simulink model "rst_auto_reg_complete_2018a"  (R2018a)
settings: Solver=VariableStepAuto  StartTime=0.0  StopTime=100  RelTol=1e-3
undefined symbols (not defined in the file): A, B, ep, initial_theta, Ta, Tas, theta_switch_time, Ts, w0
libraries: dspinverses x6, simulink x1
settings Model: Creator=tarci  LastModifiedBy=tarci

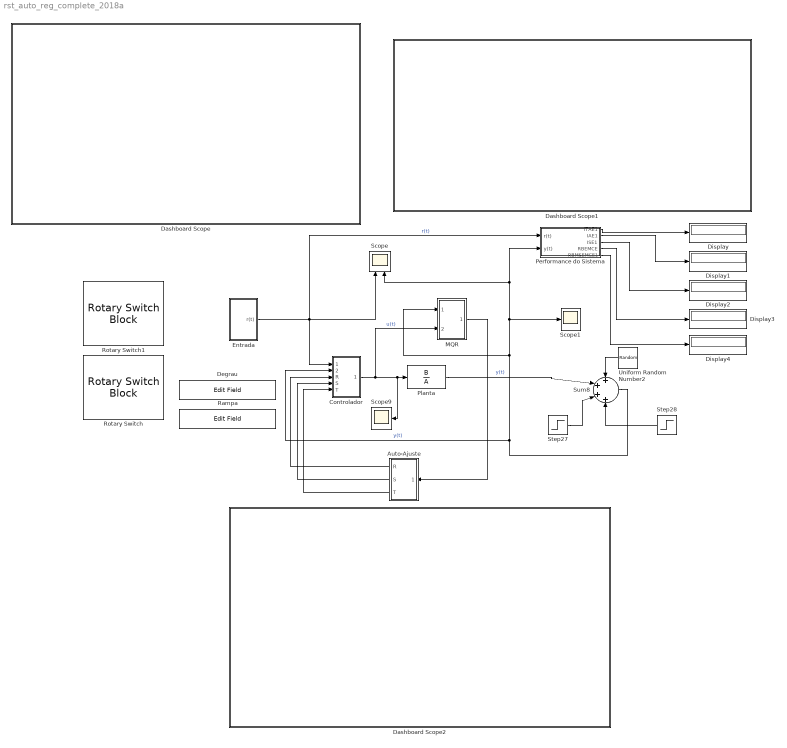
== system rst_auto_reg_complete_2018a ==
  Auto-Ajuste : Subsystem
  Controlador : Subsystem
  Dashboard Scope : Subsystem  DialogController=hmiCreateDDGDialog  IsWebBlock=on  mask(MWDashboardBlock){webBlockId=9b3c1e76-0f89-451d-9ebf-e152fc28c02b, webBlockType=sdiscope, ShowInitialText=on, HMISrcModelName=rst_auto_reg_complete_2018a}
      mask prompts: webBlockId "WebBlock Id"; webBlockType "WebBlock Type"; HMISrcModelName "Source Model"
      mask help: SimulinkHMI:dialogs:HMIScopeDialogDesc
      mask Help: helpview([docroot '/mapfiles/simulink.map'], 'hmi_scope')
      mask Display:
      | if strcmp(get_param(bdroot(gcb),'BlockDiagramType'), 'library')
      |     image([(matlabroot) '/toolbox/simulink/hmi/icons/DashboardScope.png']);
      | end
  Dashboard Scope1 : Subsystem  DialogController=hmiCreateDDGDialog  IsWebBlock=on  mask(MWDashboardBlock){webBlockId=06d563f5-1f97-498a-bfac-7182b92c07c4, webBlockType=sdiscope, ShowInitialText=on, HMISrcModelName=rst_auto_reg_complete_2018a}
      mask prompts: webBlockId "WebBlock Id"; webBlockType "WebBlock Type"; HMISrcModelName "Source Model"
      mask help: SimulinkHMI:dialogs:HMIScopeDialogDesc
      mask Help: helpview([docroot '/mapfiles/simulink.map'], 'hmi_scope')
      mask Display:
      | if strcmp(get_param(bdroot(gcb),'BlockDiagramType'), 'library')
      |     image([(matlabroot) '/toolbox/simulink/hmi/icons/DashboardScope.png']);
      | end
  Dashboard Scope2 : Subsystem  DialogController=hmiCreateDDGDialog  IsWebBlock=on  mask(MWDashboardBlock){webBlockId=9828eeca-fbfb-4c59-aa67-bf465e2bb125, webBlockType=sdiscope, ShowInitialText=on, HMISrcModelName=rst_auto_reg_complete_2018a}
      mask prompts: webBlockId "WebBlock Id"; webBlockType "WebBlock Type"; HMISrcModelName "Source Model"
      mask help: SimulinkHMI:dialogs:HMIScopeDialogDesc
      mask Help: helpview([docroot '/mapfiles/simulink.map'], 'hmi_scope')
      mask Display:
      | if strcmp(get_param(bdroot(gcb),'BlockDiagramType'), 'library')
      |     image([(matlabroot) '/toolbox/simulink/hmi/icons/DashboardScope.png']);
      | end
  Degrau : EditField  WebBlockId=626  LabelPosition=Hide  Alignment=Center
  Display{,1..4} (5 alike) : Display
  Entrada : Subsystem
  MQR : Subsystem
  Performance do Sistema : Subsystem
  Planta : DiscreteFilter  Numerator=B  Denominator=A  SampleTime=Ta  a0EqualsOne=on
  Rampa : EditField  WebBlockId=627  LabelPosition=Hide  Alignment=Center
  Rotary Switch : RotarySwitchBlock  WebBlockId=461
      settings: Values={{'Degrau', 'Rampa', 'Senoide'}, [1 2 3]}
  Rotary Switch1 : RotarySwitchBlock  WebBlockId=519
      settings: Values={{'Degrau', 'Rampa', 'Senoide'}, [1 2 3]}
  Scope : Scope  NumInputPorts=2
  Scope1 : Scope
  Scope9 : Scope
  Step27 : Step  Time=90  SampleTime=0
  Step28 : Step  Time=91  After=-1  SampleTime=0
  Sum8 : Sum  Inputs=++++
  Uniform Random Number2 : UniformRandomNumber  Minimum=-0.1  Maximum=0.1  SampleTime=0
  wires:
  Sum8/1 -> Controlador/2(y(t)), Scope1/1, Performance do Sistema/2(y(t)), Scope/2, MQR/1(y(t))  "y(t)"
  Step28/1 -> Sum8/4
  Planta/1 -> Sum8/2  "y(t)"
  Step27/1 -> Sum8/3
  Uniform Random Number2/1 -> Sum8/1
  MQR/1("Theta(t) ") -> Auto-Ajuste/1(Theta)
  Controlador/1(u(t)) -> Scope9/1, Planta/1, MQR/2("u(t) ")  "u(t)"
  Auto-Ajuste/1(R) -> Controlador/3(R)
  Auto-Ajuste/2(S) -> Controlador/4(S)
  Auto-Ajuste/3(T) -> Controlador/5(T)
  Entrada/1(r(t)) -> Performance do Sistema/1(r(t)), Scope/1, Controlador/1(r(t))  "r(t)"
  Performance do Sistema/1(ITAE1) -> Display/1
  Performance do Sistema/2(IAE1) -> Display1/1
  Performance do Sistema/3(ISE1) -> Display2/1
  Performance do Sistema/4(RBEMCE) -> Display3/1
  Performance do Sistema/5(RBMSEMCE1) -> Display4/1

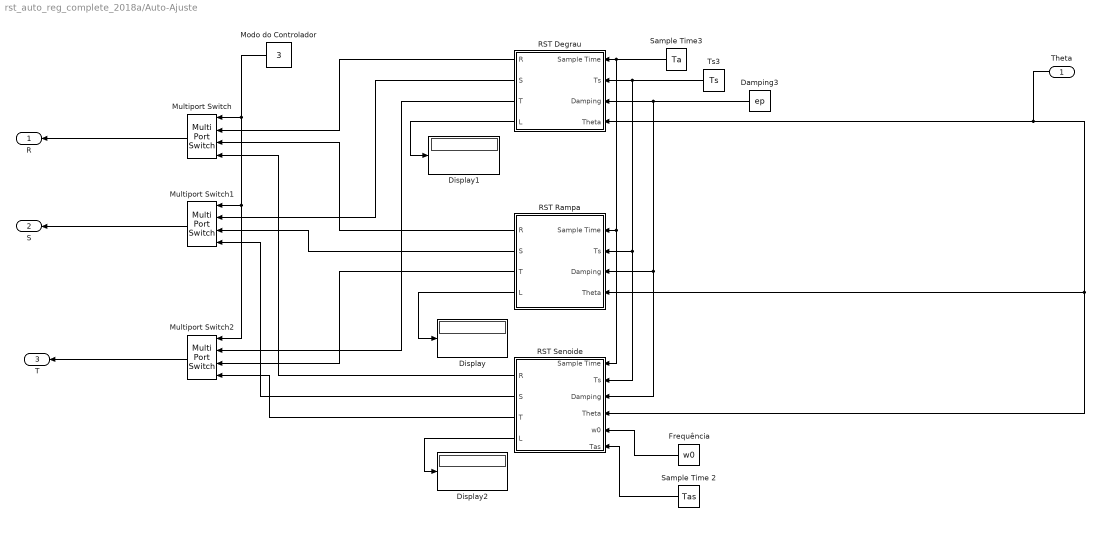
== system rst_auto_reg_complete_2018a/Auto-Ajuste ==
  Theta : Inport
  Damping3 : Constant  Value=ep
  Display : Display
  Display1 : Display
  Display2 : Display
  Frequência : Constant  Value=w0
  Modo do Controlador : Constant  Value=3
  Multiport Switch : MultiPortSwitch
  Multiport Switch1 : MultiPortSwitch
  Multiport Switch2 : MultiPortSwitch
  RST Degrau : Subsystem
  RST Rampa : Subsystem
  RST Senoide : Subsystem
  Sample Time 2 : Constant  Value=Tas
  Sample Time3 : Constant  Value=Ta
  Ts3 : Constant  Value=Ts
  R : Outport
  S : Outport  Port=2
  T : Outport  Port=3
  wires:
  Modo do Controlador/1 -> Multiport Switch2/1, Multiport Switch1/1, Multiport Switch/1
  RST Degrau/1(R) -> Multiport Switch/2
  Damping3/1 -> RST Senoide/3(Damping), RST Rampa/3(Damping), RST Degrau/3(Damping)
  RST Degrau/3(T) -> Multiport Switch2/2
  Theta/1 -> RST Senoide/4(Theta), RST Rampa/4(Theta), RST Degrau/4(Theta)
  RST Rampa/3(T) -> Multiport Switch2/3
  Sample Time3/1 -> RST Senoide/1(Sample Time), RST Rampa/1(Sample Time), RST Degrau/1(Sample Time)
  Sample Time 2/1 -> RST Senoide/6(Tas)
  Frequência/1 -> RST Senoide/5(w0)
  RST Rampa/1(R) -> Multiport Switch/3
  RST Senoide/2(S) -> Multiport Switch1/4
  RST Degrau/2(S) -> Multiport Switch1/2
  Ts3/1 -> RST Senoide/2(Ts), RST Rampa/2(Ts), RST Degrau/2(Ts)
  RST Senoide/1(R) -> Multiport Switch/4
  Multiport Switch/1 -> R/1
  Multiport Switch1/1 -> S/1
  Multiport Switch2/1 -> T/1
  RST Rampa/4(L) -> Display/1
  RST Senoide/3(T) -> Multiport Switch2/4
  RST Rampa/2(S) -> Multiport Switch1/3
  RST Degrau/4(L) -> Display1/1
  RST Senoide/4(L) -> Display2/1

== system rst_auto_reg_complete_2018a/Controlador ==
  r(t) : Inport
  y(t) : Inport  Port=2
  R : Inport  Port=3
  S : Inport  Port=4
  T : Inport  Port=5
  1/S3 : DiscreteFilter  Numerator=1  DenominatorSource=Input port  Denominator=1  SampleTime=Ta  a0EqualsOne=on
      settings: InputPortMap=u0,p3
  R3 : DiscreteFilter  NumeratorSource=Input port  Numerator=[-620.2 131.3]  Denominator=1  SampleTime=Ta
      settings: InputPortMap=u0,p1
  Sum11 : Sum  Inputs=|+-
  T3 : DiscreteFilter  NumeratorSource=Input port  Numerator=13.39  Denominator=1  SampleTime=Ta
      settings: InputPortMap=u0,p1
  u(t) : Outport
  wires:
  T3/1 -> Sum11/1
  T/1 -> T3/2  "T"
  Sum11/1 -> 1/S3/1
  R3/1 -> Sum11/2
  R/1 -> R3/2
  S/1 -> 1/S3/2
  r(t)/1 -> T3/1
  y(t)/1 -> R3/1
  1/S3/1 -> u(t)/1  "u(t)"

== system rst_auto_reg_complete_2018a/Dashboard Scope ==

== system rst_auto_reg_complete_2018a/Dashboard Scope1 ==

== system rst_auto_reg_complete_2018a/Dashboard Scope2 ==

== system rst_auto_reg_complete_2018a/Entrada ==
  Multiport Switch : MultiPortSwitch
  Ramp : simulink/Sources/Ramp  slope=1  start=0  InitialOutput=0
  Sine Wave : Sin  Frequency=w0  SampleTime=Tas
  Step1 : Step  Time=0  After=2  SampleTime=0
  Tipo de Entrada : Constant  Value=3
  r(t) : Outport
  wires:
  Sine Wave/1 -> Multiport Switch/4
  Step1/1 -> Multiport Switch/2
  Ramp/1 -> Multiport Switch/3
  Tipo de Entrada/1 -> Multiport Switch/1
  Multiport Switch/1 -> r(t)/1

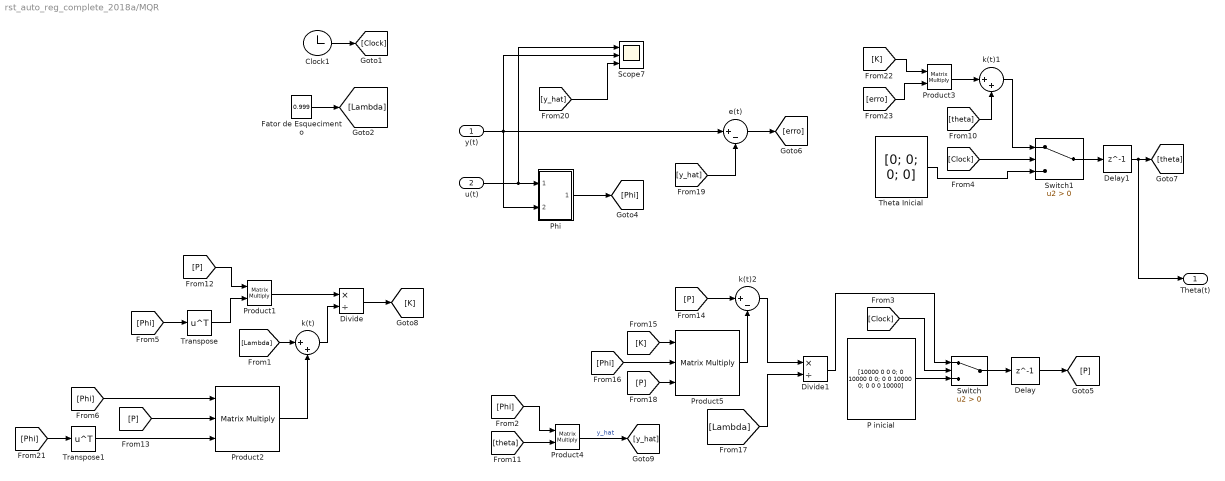
== system rst_auto_reg_complete_2018a/MQR ==
  y(t) : Inport
  "u(t) " : Inport  Port=2
  Clock1 : Clock
  Delay : Delay  DelayLength=1  InitialCondition=0
  Delay1 : Delay  DelayLength=1  InitialCondition=0
  Divide : Product  Inputs=*/
  Divide1 : Product  Inputs=*/
  "Fator de Esquecimento " : Constant  Value=0.999
  P inicial : Constant  Value=[10000 0 0 0; 0 10000 0 0; 0 0 10000 0; 0 0 0 10000]
  Phi : Subsystem
  Product1 : Product  Multiplication=Matrix(*)
  Product2 : Product  Inputs=3  Multiplication=Matrix(*)
  Product3 : Product  Multiplication=Matrix(*)
  Product4 : Product  Multiplication=Matrix(*)
  Product5 : Product  Inputs=3  Multiplication=Matrix(*)
  Scope7 : Scope  NumInputPorts=3
  Switch : Switch  Criteria=u2 > Threshold
  Switch1 : Switch  Criteria=u2 > Threshold
  "Theta Inicial " : Constant  Value=[0; 0; 0; 0]
  Transpose : Math  Operator=transpose  SaturateOnIntegerOverflow=on
  Transpose1 : Math  Operator=transpose  SaturateOnIntegerOverflow=on
  e(t) : Sum  Inputs=|+-
  k(t) : Sum  Inputs=|++
  k(t)1 : Sum  Inputs=|++
  k(t)2 : Sum  Inputs=|+-
  "Theta(t) " : Outport
  wires:
  k(t)/1 -> Divide/2
  [Phi] -> Product4/1
  Phi/1(Phi) -> [Phi]
  k(t)1/1 -> Switch1/1
  [y_hat] -> Scope7/3
  Switch1/1 -> Delay1/1
  [K] -> Product3/1
  Product2/1 -> k(t)/2
  [Clock] -> Switch1/2
  y(t)/1 -> e(t)/1, Scope7/2, Phi/2(y(t))
  k(t)2/1 -> Divide1/1
  Delay1/1 -> "Theta(t) "/1, [theta]
  Product5/1 -> k(t)2/2
  "u(t) "/1 -> Scope7/1, Phi/1(u(t))
  Switch/1 -> Delay/1
  [Lambda] -> Divide1/2
  Product1/1 -> Divide/1
  e(t)/1 -> [erro]
  Product3/1 -> k(t)1/1
  Delay/1 -> [P]
  [Phi] -> Transpose1/1
  [P] -> Product5/3
  "Fator de Esquecimento "/1 -> [Lambda]
  "Theta Inicial "/1 -> Switch1/3
  Transpose1/1 -> Product2/3
  Divide1/1 -> Switch/1
  [Phi] -> Transpose/1
  [Clock] -> Switch/2
  [theta] -> Product4/2
  [P] -> k(t)2/1
  [theta] -> k(t)1/2
  [P] -> Product2/2
  [Lambda] -> k(t)/1
  Transpose/1 -> Product1/2
  Clock1/1 -> [Clock]
  [erro] -> Product3/2
  [y_hat] -> e(t)/2
  [K] -> Product5/1
  P inicial/1 -> Switch/3
  [P] -> Product1/1
  [Phi] -> Product2/1
  Divide/1 -> [K]
  [Phi] -> Product5/2
  Product4/1 -> [y_hat]  "y_hat"

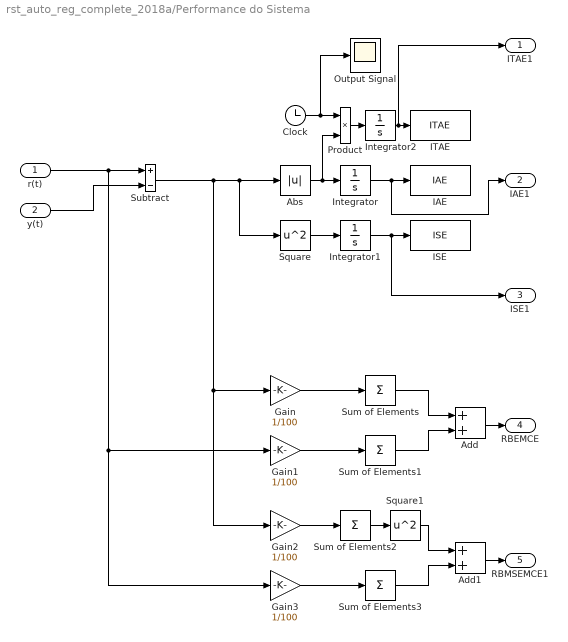
== system rst_auto_reg_complete_2018a/Performance do Sistema ==
  r(t) : Inport
  y(t) : Inport  Port=2
  Abs : Abs
  Add : Sum
  Add1 : Sum
  Clock : Clock
  Gain{,1..3} (4 alike) : Gain  Gain=1/100
  IAE : ToWorkspace  VariableName=IAE  SaveFormat=Timeseries  SampleTime=-1
  ISE : ToWorkspace  VariableName=ISE  SaveFormat=Timeseries  SampleTime=-1
  ITAE : ToWorkspace  VariableName=ITAE  SaveFormat=Timeseries  SampleTime=-1
  Integrator : Integrator
  Integrator1 : Integrator
  Integrator2 : Integrator
  Output Signal : Scope
  Product : Product
  Square : Math  Operator=square  SaturateOnIntegerOverflow=on
  Square1 : Math  Operator=square  SaturateOnIntegerOverflow=on
  Subtract : Sum  Inputs=+-
  Sum of Elements{,1..3} (4 alike) : Sum  Inputs=+
  ITAE1 : Outport
  IAE1 : Outport  Port=2
  ISE1 : Outport  Port=3
  RBEMCE : Outport  Port=4
  RBMSEMCE1 : Outport  Port=5
  wires:
  y(t)/1 -> Subtract/2
  Abs/1 -> Product/2, Integrator/1
  Integrator/1 -> IAE1/1, IAE/1
  Integrator1/1 -> ISE1/1, ISE/1
  Square/1 -> Integrator1/1
  Clock/1 -> Output Signal/1, Product/1
  Product/1 -> Integrator2/1
  Integrator2/1 -> ITAE1/1, ITAE/1
  Gain/1 -> Sum of Elements/1
  Gain1/1 -> Sum of Elements1/1
  Sum of Elements/1 -> Add/1
  Sum of Elements1/1 -> Add/2
  Add/1 -> RBEMCE/1
  Add1/1 -> RBMSEMCE1/1
  Sum of Elements3/1 -> Add1/2
  Sum of Elements2/1 -> Square1/1
  Gain3/1 -> Sum of Elements3/1
  Gain2/1 -> Sum of Elements2/1
  r(t)/1 -> Gain3/1, Gain1/1, Subtract/1
  Subtract/1 -> Gain2/1, Gain/1, Square/1, Abs/1
  Square1/1 -> Add1/1

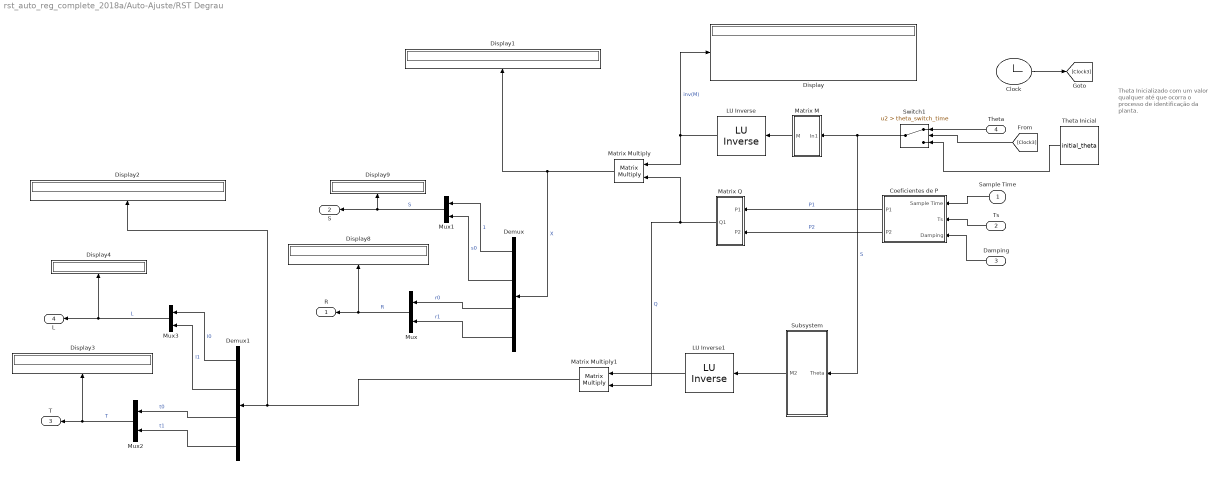
== system rst_auto_reg_complete_2018a/Auto-Ajuste/RST Degrau ==
  note: Theta Inicializado com um
      | valor qualquer até que ocorra
      |  o processo de identificação
      | da planta.
  Sample Time : Inport
  Ts : Inport  Port=2
  Damping : Inport  Port=3
  Theta : Inport  Port=4
  " LU Inverse" : dspinverses/ LU Inverse
      settings: SourceProductName=DSP System Toolbox
  " LU Inverse1" : dspinverses/ LU Inverse
      settings: SourceProductName=DSP System Toolbox
  Clock : Clock
  Coeficientes de P : Subsystem
  Demux : Demux
  Demux1 : Demux
  Display{,1..4,8..9} (7 alike) : Display
  Matrix M : Subsystem
  Matrix Multiply : Product  Multiplication=Matrix(*)
  Matrix Multiply1 : Product  Multiplication=Matrix(*)
  Matrix Q : Subsystem
  Mux{,1..3} (4 alike) : Mux  Inputs=2
  Subsystem : Subsystem
  Switch1 : Switch  Criteria=u2 > Threshold  Threshold=theta_switch_time
  Theta Inicial : Constant  Value=initial_theta
  R : Outport
  S : Outport  Port=2
  T : Outport  Port=3
  L : Outport  Port=4
  wires:
  Matrix Multiply/1 -> Demux/1, Display1/1  "X"
  " LU Inverse"/1 -> Matrix Multiply/1, Display/1  "inv(M)"
  Mux1/1 -> S/1, Display9/1  "S"
  Coeficientes de P/2(P2) -> Matrix Q/2(P2)  "P2"
  Ts/1 -> Coeficientes de P/2(Ts)
  Damping/1 -> Coeficientes de P/3(Damping)
  Sample Time/1 -> Coeficientes de P/1(Sample Time)
  Coeficientes de P/1(P1) -> Matrix Q/1(P1)  "P1"
  Mux/1 -> R/1, Display8/1  "R"
  Clock/1 -> [Clock3]
  Switch1/1 -> Subsystem/1(Theta), Matrix M/1(In1)  "S"
  Theta/1 -> Switch1/1
  [Clock3] -> Switch1/2
  Theta Inicial/1 -> Switch1/3
  Matrix M/1(M) -> " LU Inverse"/1
  Demux/1 -> Mux1/1  "1"
  Demux/2 -> Mux1/2  "s0"
  Demux/3 -> Mux/1  "r0"
  Demux/4 -> Mux/2  "r1"
  " LU Inverse1"/1 -> Matrix Multiply1/1
  Matrix Q/1(Q1) -> Matrix Multiply1/2, Matrix Multiply/2  "Q"
  Subsystem/1(M2) -> " LU Inverse1"/1
  Demux1/3 -> Mux2/1  "t0"
  Mux2/1 -> T/1, Display3/1  "T"
  Demux1/2 -> Mux3/2  "l1"
  Mux3/1 -> L/1, Display4/1  "L"
  Demux1/1 -> Mux3/1  "l0"
  Matrix Multiply1/1 -> Display2/1, Demux1/1
  Demux1/4 -> Mux2/2  "t1"

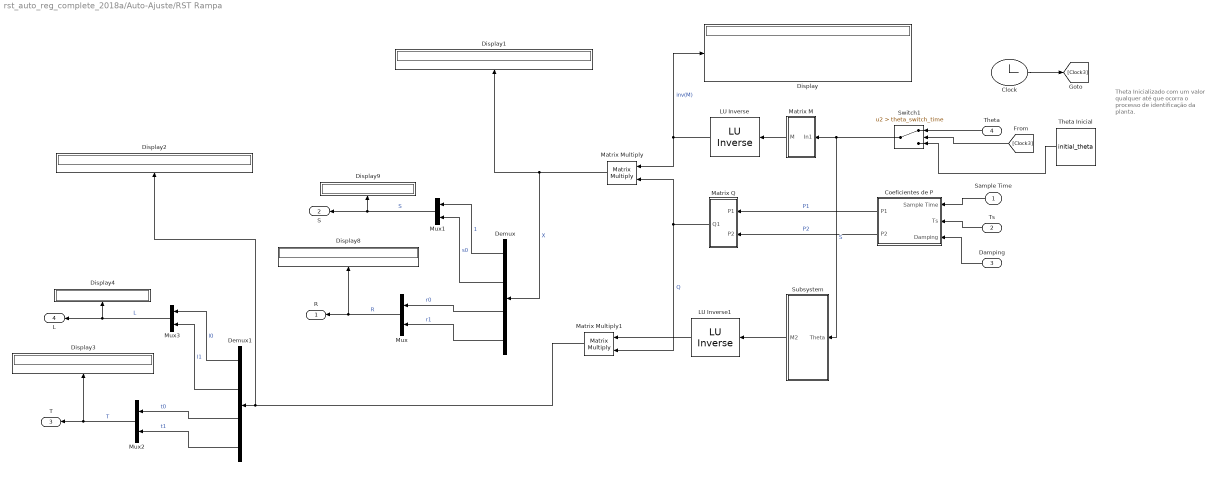
== system rst_auto_reg_complete_2018a/Auto-Ajuste/RST Rampa ==
  note: Theta Inicializado com um
      | valor qualquer até que ocorra
      |  o processo de identificação
      | da planta.
  Sample Time : Inport
  Ts : Inport  Port=2
  Damping : Inport  Port=3
  Theta : Inport  Port=4
  " LU Inverse" : dspinverses/ LU Inverse
      settings: SourceProductName=DSP System Toolbox
  " LU Inverse1" : dspinverses/ LU Inverse
      settings: SourceProductName=DSP System Toolbox
  Clock : Clock
  Coeficientes de P : Subsystem
  Demux : Demux
  Demux1 : Demux
  Display{,1..4,8..9} (7 alike) : Display
  Matrix M : Subsystem
  Matrix Multiply : Product  Multiplication=Matrix(*)
  Matrix Multiply1 : Product  Multiplication=Matrix(*)
  Matrix Q : Subsystem
  Mux{,1..3} (4 alike) : Mux  Inputs=2
  Subsystem : Subsystem
  Switch1 : Switch  Criteria=u2 > Threshold  Threshold=theta_switch_time
  Theta Inicial : Constant  Value=initial_theta
  R : Outport
  S : Outport  Port=2
  T : Outport  Port=3
  L : Outport  Port=4
  wires:
  Demux/4 -> Mux/2  "r1"
  Demux/3 -> Mux/1  "r0"
  Demux/2 -> Mux1/2  "s0"
  Demux/1 -> Mux1/1  "1"
  Matrix Q/1(Q1) -> Matrix Multiply1/2, Matrix Multiply/2  "Q"
  Matrix M/1(M) -> " LU Inverse"/1
  Theta Inicial/1 -> Switch1/3
  [Clock3] -> Switch1/2
  Theta/1 -> Switch1/1
  Switch1/1 -> Subsystem/1(Theta), Matrix M/1(In1)  "S"
  Clock/1 -> [Clock3]
  Mux/1 -> Display8/1, R/1  "R"
  Coeficientes de P/1(P1) -> Matrix Q/1(P1)  "P1"
  Sample Time/1 -> Coeficientes de P/1(Sample Time)
  Damping/1 -> Coeficientes de P/3(Damping)
  Ts/1 -> Coeficientes de P/2(Ts)
  Coeficientes de P/2(P2) -> Matrix Q/2(P2)  "P2"
  Mux1/1 -> Display9/1, S/1  "S"
  " LU Inverse"/1 -> Display/1, Matrix Multiply/1  "inv(M)"
  Matrix Multiply/1 -> Display1/1, Demux/1  "X"
  Subsystem/1(M2) -> " LU Inverse1"/1
  " LU Inverse1"/1 -> Matrix Multiply1/1
  Mux3/1 -> L/1, Display4/1  "L"
  Mux2/1 -> T/1, Display3/1  "T"
  Demux1/1 -> Mux3/1  "l0"
  Demux1/2 -> Mux3/2  "l1"
  Demux1/3 -> Mux2/1  "t0"
  Demux1/4 -> Mux2/2  "t1"
  Matrix Multiply1/1 -> Display2/1, Demux1/1

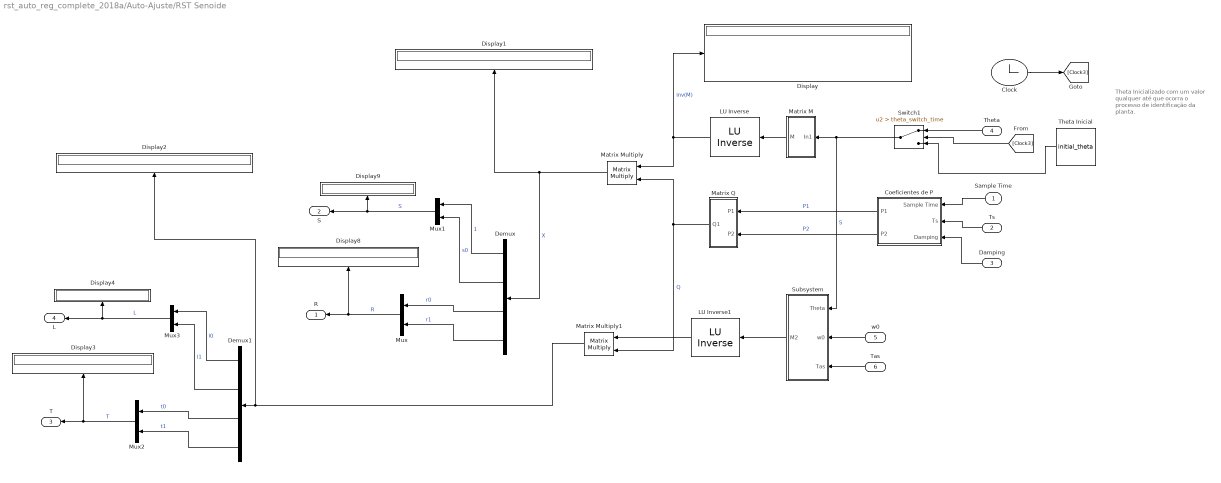
== system rst_auto_reg_complete_2018a/Auto-Ajuste/RST Senoide ==
  note: Theta Inicializado com um
      | valor qualquer até que ocorra
      |  o processo de identificação
      | da planta.
  Sample Time : Inport
  Ts : Inport  Port=2
  Damping : Inport  Port=3
  Theta : Inport  Port=4
  w0 : Inport  Port=5
  Tas : Inport  Port=6
  " LU Inverse" : dspinverses/ LU Inverse
      settings: SourceProductName=DSP System Toolbox
  " LU Inverse1" : dspinverses/ LU Inverse
      settings: SourceProductName=DSP System Toolbox
  Clock : Clock
  Coeficientes de P : Subsystem
  Demux : Demux
  Demux1 : Demux
  Display{,1..4,8..9} (7 alike) : Display
  Matrix M : Subsystem
  Matrix Multiply : Product  Multiplication=Matrix(*)
  Matrix Multiply1 : Product  Multiplication=Matrix(*)
  Matrix Q : Subsystem
  Mux{,1..3} (4 alike) : Mux  Inputs=2
  Subsystem : Subsystem
  Switch1 : Switch  Criteria=u2 > Threshold  Threshold=theta_switch_time
  Theta Inicial : Constant  Value=initial_theta
  R : Outport
  S : Outport  Port=2
  T : Outport  Port=3
  L : Outport  Port=4
  wires:
  Demux/4 -> Mux/2  "r1"
  Demux/3 -> Mux/1  "r0"
  Demux/2 -> Mux1/2  "s0"
  Demux/1 -> Mux1/1  "1"
  Matrix Q/1(Q1) -> Matrix Multiply1/2, Matrix Multiply/2  "Q"
  Matrix M/1(M) -> " LU Inverse"/1
  Theta Inicial/1 -> Switch1/3
  [Clock3] -> Switch1/2
  Theta/1 -> Switch1/1
  Switch1/1 -> Subsystem/1(Theta), Matrix M/1(In1)  "S"
  Clock/1 -> [Clock3]
  Mux/1 -> Display8/1, R/1  "R"
  Coeficientes de P/1(P1) -> Matrix Q/1(P1)  "P1"
  Sample Time/1 -> Coeficientes de P/1(Sample Time)
  Damping/1 -> Coeficientes de P/3(Damping)
  Ts/1 -> Coeficientes de P/2(Ts)
  Coeficientes de P/2(P2) -> Matrix Q/2(P2)  "P2"
  Mux1/1 -> Display9/1, S/1  "S"
  " LU Inverse"/1 -> Display/1, Matrix Multiply/1  "inv(M)"
  Matrix Multiply/1 -> Display1/1, Demux/1  "X"
  w0/1 -> Subsystem/2(w0)
  Tas/1 -> Subsystem/3(Tas)
  Subsystem/1(M2) -> " LU Inverse1"/1
  " LU Inverse1"/1 -> Matrix Multiply1/1
  Mux3/1 -> L/1, Display4/1  "L"
  Mux2/1 -> T/1, Display3/1  "T"
  Demux1/1 -> Mux3/1  "l0"
  Demux1/2 -> Mux3/2  "l1"
  Demux1/3 -> Mux2/1  "t0"
  Demux1/4 -> Mux2/2  "t1"
  Matrix Multiply1/1 -> Display2/1, Demux1/1

== system rst_auto_reg_complete_2018a/MQR/Phi ==
  u(t) : Inport
  y(t) : Inport  Port=2
  Constant : Constant  Value=-1
  Delay : Delay
  Delay1 : Delay  DelayLength=1
  Delay2 : Delay
  Delay3 : Delay  DelayLength=1
  Display : Display
  Product : Product
  Transpose1 : Math  Operator=transpose  SaturateOnIntegerOverflow=on
  Vector Concatenate : Concatenate  NumInputs=4
  Phi : Outport
  wires:
  u(t)/1 -> Delay2/1, Delay3/1
  Vector Concatenate/1 -> Transpose1/1, Display/1  "Phi"
  Delay/1 -> Vector Concatenate/2
  y(t)/1 -> Product/1
  Delay3/1 -> Vector Concatenate/3
  Delay2/1 -> Vector Concatenate/4
  Delay1/1 -> Vector Concatenate/1
  Transpose1/1 -> Phi/1
  Constant/1 -> Product/2
  Product/1 -> Delay/1, Delay1/1

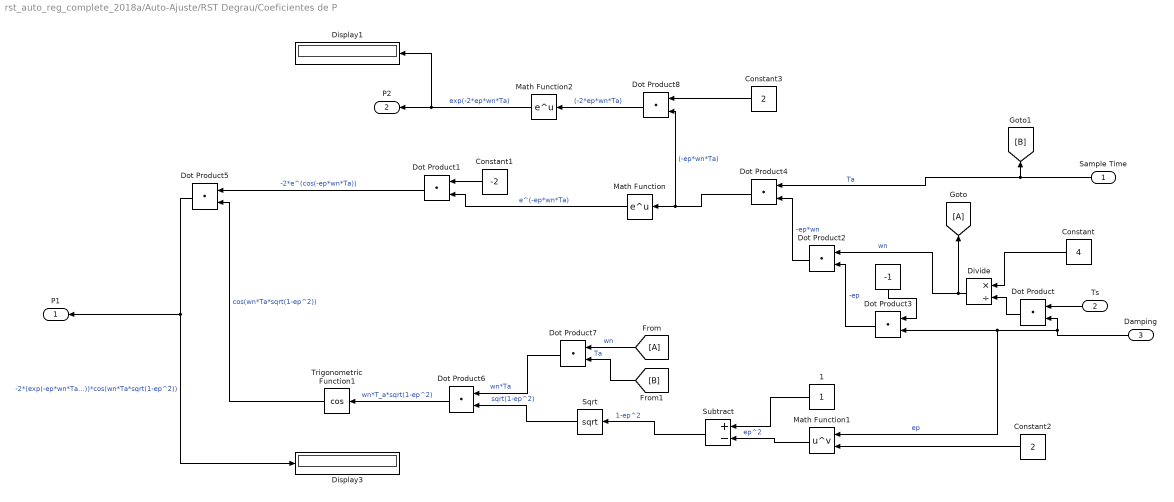
== system rst_auto_reg_complete_2018a/Auto-Ajuste/RST Degrau/Coeficientes de P ==
  Sample Time : Inport
  Ts : Inport  Port=2
  Damping : Inport  Port=3
  " " : Constant  Value=-1
  1 : Constant
  Constant : Constant  Value=4
  Constant1 : Constant  Value=-2
  Constant2 : Constant  Value=2
  Constant3 : Constant  Value=2
  Display1 : Display
  Display3 : Display
  Divide : Product  Inputs=*/
  Dot Product{,1..8} (9 alike) : DotProduct  InputSameDT=on  OutDataTypeStr=Inherit: Inherit via internal rule
  Math Function : Math  SaturateOnIntegerOverflow=on
  Math Function1 : Math  Operator=pow  SaturateOnIntegerOverflow=on
  Math Function2 : Math  SaturateOnIntegerOverflow=on
  Sqrt : Sqrt  SaturateOnIntegerOverflow=on
  Subtract : Sum  Inputs=+-
  Trigonometric Function1 : Trigonometry  Operator=cos
  P1 : Outport
  P2 : Outport  Port=2
  wires:
  Math Function/1 -> Dot Product1/2  "e^(-ep*wn*Ta)"
  Divide/1 -> [A], Dot Product2/1  "wn"
  [A] -> Dot Product7/1  "wn"
  " "/1 -> Dot Product3/1
  Dot Product5/1 -> P1/1, Display3/1  "-2*(exp(-ep*wn*Ta))*cos(wn*Ta*sqrt(1-ep^2))"
  Trigonometric Function1/1 -> Dot Product5/2  "cos(wn*Ta*sqrt(1-ep^2))"
  Ts/1 -> Dot Product/1
  Dot Product/1 -> Divide/2
  Dot Product3/1 -> Dot Product2/2  "-ep"
  Damping/1 -> Math Function1/1, Dot Product3/2, Dot Product/2  "ep"
  Constant/1 -> Divide/1
  Dot Product7/1 -> Dot Product6/1  "wn*Ta"
  Sample Time/1 -> Dot Product4/1, [B]  "Ta"
  Math Function1/1 -> Subtract/2  "ep^2"
  Dot Product1/1 -> Dot Product5/1  "-2*e^(cos(-ep*wn*Ta))"
  Constant2/1 -> Math Function1/2
  1/1 -> Subtract/1
  Constant1/1 -> Dot Product1/1
  Dot Product2/1 -> Dot Product4/2  "-ep*wn"
  [B] -> Dot Product7/2  "Ta"
  Dot Product6/1 -> Trigonometric Function1/1  "wn*T_a*sqrt(1-ep^2)"
  Dot Product4/1 -> Dot Product8/2, Math Function/1  "(-ep*wn*Ta)"
  Sqrt/1 -> Dot Product6/2  "sqrt(1-ep^2)"
  Subtract/1 -> Sqrt/1  "1-ep^2"
  Constant3/1 -> Dot Product8/1
  Dot Product8/1 -> Math Function2/1  "(-2*ep*wn*Ta)"
  Math Function2/1 -> Display1/1, P2/1  "exp(-2*ep*wn*Ta)"

== system rst_auto_reg_complete_2018a/Auto-Ajuste/RST Degrau/Matrix M ==
  In1 : Inport
  " 1" : Constant  Value=0
  2 : Constant
  Demux : Demux
  Display1 : Display
  Matrix Concatenate{6,9..11} (4 alike) : Concatenate  NumInputs=4  Mode=Multidimensional array  ConcatenateDimension=2
  Matrix Concatenate12 : Concatenate  Mode=Multidimensional array
  Matrix Concatenate13 : Concatenate  Mode=Multidimensional array
  Matrix Concatenate14 : Concatenate  Mode=Multidimensional array
  M : Outport
  wires:
  In1/1 -> Demux/1
  Demux/3 -> Matrix Concatenate9/3, Matrix Concatenate10/4  "b1"
  Matrix Concatenate14/1 -> M/1, Display1/1
  Demux/1 -> Matrix Concatenate10/2, Matrix Concatenate9/1  "a1"
  Demux/4 -> Matrix Concatenate11/4, Matrix Concatenate10/3  "b2"
  Demux/2 -> Matrix Concatenate11/2, Matrix Concatenate10/1  "a2"
  2/1 -> Matrix Concatenate9/2, Matrix Concatenate6/1  "1"
  " 1"/1 -> Matrix Concatenate6/3, Matrix Concatenate11/3, Matrix Concatenate11/1, Matrix Concatenate9/4, Matrix Concatenate6/4, Matrix Concatenate6/2  "0"
  Matrix Concatenate6/1 -> Matrix Concatenate12/1
  Matrix Concatenate9/1 -> Matrix Concatenate12/2
  Matrix Concatenate10/1 -> Matrix Concatenate13/1
  Matrix Concatenate11/1 -> Matrix Concatenate13/2
  Matrix Concatenate13/1 -> Matrix Concatenate14/2
  Matrix Concatenate12/1 -> Matrix Concatenate14/1

== system rst_auto_reg_complete_2018a/Auto-Ajuste/RST Degrau/Matrix Q ==
  P1 : Inport
  P2 : Inport  Port=2
  Constant : Constant
  Constant1 : Constant  Value=0
  Display1 : Display
  Matrix Concatenate1 : Concatenate  Mode=Multidimensional array
  Matrix Concatenate2 : Concatenate  Mode=Multidimensional array
  Matrix Concatenate3 : Concatenate  Mode=Multidimensional array
  Q1 : Outport
  wires:
  Matrix Concatenate1/1 -> Matrix Concatenate2/1
  Matrix Concatenate2/1 -> Q1/1, Display1/1
  Matrix Concatenate3/1 -> Matrix Concatenate2/2
  P2/1 -> Matrix Concatenate3/1
  P1/1 -> Matrix Concatenate1/2
  Constant/1 -> Matrix Concatenate1/1
  Constant1/1 -> Matrix Concatenate3/2

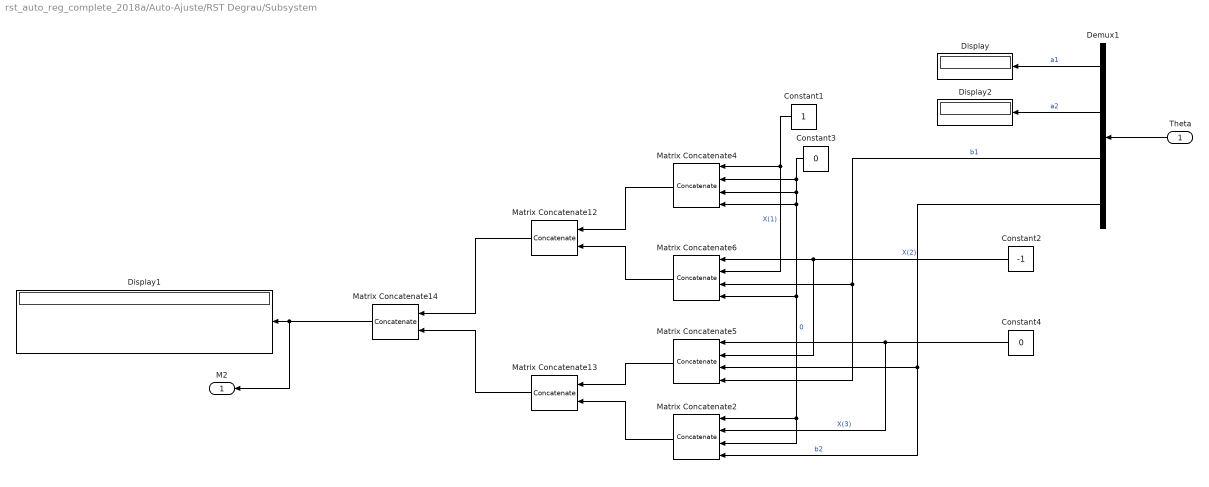
== system rst_auto_reg_complete_2018a/Auto-Ajuste/RST Degrau/Subsystem ==
  Theta : Inport
  Constant1 : Constant
  Constant2 : Constant  Value=-1
  Constant3 : Constant  Value=0
  Constant4 : Constant  Value=0
  Demux1 : Demux
  Display : Display
  Display1 : Display
  Display2 : Display
  Matrix Concatenate12 : Concatenate  Mode=Multidimensional array
  Matrix Concatenate13 : Concatenate  Mode=Multidimensional array
  Matrix Concatenate14 : Concatenate  Mode=Multidimensional array
  Matrix Concatenate{2,4..6} (4 alike) : Concatenate  NumInputs=4  Mode=Multidimensional array  ConcatenateDimension=2
  M2 : Outport
  wires:
  Matrix Concatenate6/1 -> Matrix Concatenate12/2
  Demux1/2 -> Display2/1  "a2"
  Theta/1 -> Demux1/1
  Demux1/1 -> Display/1  "a1"
  Constant1/1 -> Matrix Concatenate6/2, Matrix Concatenate4/1  "X(1)"
  Constant3/1 -> Matrix Concatenate4/3, Matrix Concatenate2/3, Matrix Concatenate2/1, Matrix Concatenate6/4, Matrix Concatenate4/4, Matrix Concatenate4/2  "0"
  Demux1/3 -> Matrix Concatenate5/4, Matrix Concatenate6/3  "b1"
  Demux1/4 -> Matrix Concatenate2/4, Matrix Concatenate5/3  "b2"
  Matrix Concatenate14/1 -> Display1/1, M2/1
  Matrix Concatenate13/1 -> Matrix Concatenate14/2
  Matrix Concatenate12/1 -> Matrix Concatenate14/1
  Matrix Concatenate4/1 -> Matrix Concatenate12/1
  Matrix Concatenate5/1 -> Matrix Concatenate13/1
  Matrix Concatenate2/1 -> Matrix Concatenate13/2
  Constant2/1 -> Matrix Concatenate5/2, Matrix Concatenate6/1  "X(2)"
  Constant4/1 -> Matrix Concatenate2/2, Matrix Concatenate5/1  "X(3)"

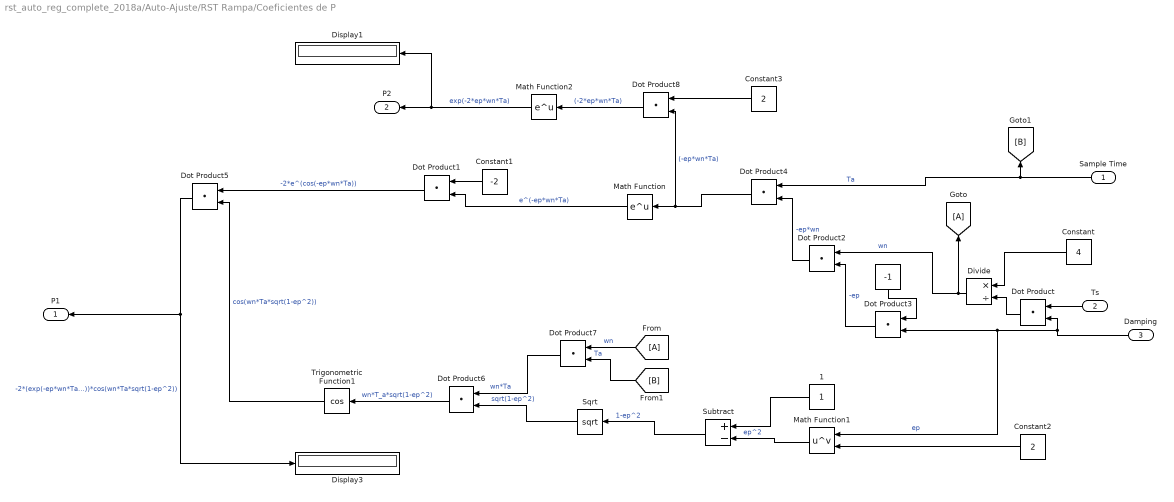
== system rst_auto_reg_complete_2018a/Auto-Ajuste/RST Rampa/Coeficientes de P ==
  Sample Time : Inport
  Ts : Inport  Port=2
  Damping : Inport  Port=3
  " " : Constant  Value=-1
  1 : Constant
  Constant : Constant  Value=4
  Constant1 : Constant  Value=-2
  Constant2 : Constant  Value=2
  Constant3 : Constant  Value=2
  Display1 : Display
  Display3 : Display
  Divide : Product  Inputs=*/
  Dot Product{,1..8} (9 alike) : DotProduct  InputSameDT=on  OutDataTypeStr=Inherit: Inherit via internal rule
  Math Function : Math  SaturateOnIntegerOverflow=on
  Math Function1 : Math  Operator=pow  SaturateOnIntegerOverflow=on
  Math Function2 : Math  SaturateOnIntegerOverflow=on
  Sqrt : Sqrt  SaturateOnIntegerOverflow=on
  Subtract : Sum  Inputs=+-
  Trigonometric Function1 : Trigonometry  Operator=cos
  P1 : Outport
  P2 : Outport  Port=2
  wires:
  Math Function2/1 -> P2/1, Display1/1  "exp(-2*ep*wn*Ta)"
  Dot Product8/1 -> Math Function2/1  "(-2*ep*wn*Ta)"
  Constant3/1 -> Dot Product8/1
  Subtract/1 -> Sqrt/1  "1-ep^2"
  Sqrt/1 -> Dot Product6/2  "sqrt(1-ep^2)"
  Dot Product4/1 -> Math Function/1, Dot Product8/2  "(-ep*wn*Ta)"
  Dot Product6/1 -> Trigonometric Function1/1  "wn*T_a*sqrt(1-ep^2)"
  [B] -> Dot Product7/2  "Ta"
  Dot Product2/1 -> Dot Product4/2  "-ep*wn"
  Constant1/1 -> Dot Product1/1
  1/1 -> Subtract/1
  Constant2/1 -> Math Function1/2
  Dot Product1/1 -> Dot Product5/1  "-2*e^(cos(-ep*wn*Ta))"
  Math Function1/1 -> Subtract/2  "ep^2"
  Sample Time/1 -> [B], Dot Product4/1  "Ta"
  Dot Product7/1 -> Dot Product6/1  "wn*Ta"
  Constant/1 -> Divide/1
  Damping/1 -> Dot Product/2, Dot Product3/2, Math Function1/1  "ep"
  Dot Product3/1 -> Dot Product2/2  "-ep"
  Dot Product/1 -> Divide/2
  Ts/1 -> Dot Product/1
  Trigonometric Function1/1 -> Dot Product5/2  "cos(wn*Ta*sqrt(1-ep^2))"
  Dot Product5/1 -> Display3/1, P1/1  "-2*(exp(-ep*wn*Ta))*cos(wn*Ta*sqrt(1-ep^2))"
  " "/1 -> Dot Product3/1
  [A] -> Dot Product7/1  "wn"
  Divide/1 -> Dot Product2/1, [A]  "wn"
  Math Function/1 -> Dot Product1/2  "e^(-ep*wn*Ta)"

== system rst_auto_reg_complete_2018a/Auto-Ajuste/RST Rampa/Matrix M ==
  In1 : Inport
  " 1" : Constant  Value=0
  2 : Constant
  Demux : Demux
  Display1 : Display
  Matrix Concatenate{6,9..11} (4 alike) : Concatenate  NumInputs=4  Mode=Multidimensional array  ConcatenateDimension=2
  Matrix Concatenate12 : Concatenate  Mode=Multidimensional array
  Matrix Concatenate13 : Concatenate  Mode=Multidimensional array
  Matrix Concatenate14 : Concatenate  Mode=Multidimensional array
  M : Outport
  wires:
  Matrix Concatenate12/1 -> Matrix Concatenate14/1
  Matrix Concatenate13/1 -> Matrix Concatenate14/2
  Matrix Concatenate11/1 -> Matrix Concatenate13/2
  Matrix Concatenate10/1 -> Matrix Concatenate13/1
  Matrix Concatenate9/1 -> Matrix Concatenate12/2
  Matrix Concatenate6/1 -> Matrix Concatenate12/1
  " 1"/1 -> Matrix Concatenate6/2, Matrix Concatenate6/4, Matrix Concatenate9/4, Matrix Concatenate11/1, Matrix Concatenate11/3, Matrix Concatenate6/3  "0"
  2/1 -> Matrix Concatenate6/1, Matrix Concatenate9/2  "1"
  Demux/2 -> Matrix Concatenate10/1, Matrix Concatenate11/2  "a2"
  Demux/4 -> Matrix Concatenate10/3, Matrix Concatenate11/4  "b2"
  Demux/1 -> Matrix Concatenate9/1, Matrix Concatenate10/2  "a1"
  Matrix Concatenate14/1 -> Display1/1, M/1
  Demux/3 -> Matrix Concatenate10/4, Matrix Concatenate9/3  "b1"
  In1/1 -> Demux/1

== system rst_auto_reg_complete_2018a/Auto-Ajuste/RST Rampa/Matrix Q ==
  P1 : Inport
  P2 : Inport  Port=2
  Constant : Constant
  Constant1 : Constant  Value=0
  Display1 : Display
  Matrix Concatenate1 : Concatenate  Mode=Multidimensional array
  Matrix Concatenate2 : Concatenate  Mode=Multidimensional array
  Matrix Concatenate3 : Concatenate  Mode=Multidimensional array
  Q1 : Outport
  wires:
  Constant1/1 -> Matrix Concatenate3/2
  Constant/1 -> Matrix Concatenate1/1
  P1/1 -> Matrix Concatenate1/2
  P2/1 -> Matrix Concatenate3/1
  Matrix Concatenate3/1 -> Matrix Concatenate2/2
  Matrix Concatenate2/1 -> Display1/1, Q1/1
  Matrix Concatenate1/1 -> Matrix Concatenate2/1

== system rst_auto_reg_complete_2018a/Auto-Ajuste/RST Rampa/Subsystem ==
  Theta : Inport
  Constant1 : Constant
  Constant2 : Constant  Value=-2
  Constant3 : Constant  Value=0
  Constant4 : Constant
  Demux1 : Demux
  Display : Display
  Display1 : Display
  Display2 : Display
  Matrix Concatenate12 : Concatenate  Mode=Multidimensional array
  Matrix Concatenate13 : Concatenate  Mode=Multidimensional array
  Matrix Concatenate14 : Concatenate  Mode=Multidimensional array
  Matrix Concatenate{2,4..6} (4 alike) : Concatenate  NumInputs=4  Mode=Multidimensional array  ConcatenateDimension=2
  M2 : Outport
  wires:
  Matrix Concatenate6/1 -> Matrix Concatenate12/2
  Demux1/2 -> Display2/1  "a2"
  Theta/1 -> Demux1/1
  Demux1/1 -> Display/1  "a1"
  Constant1/1 -> Matrix Concatenate6/2, Matrix Concatenate4/1  "X(1)"
  Constant3/1 -> Matrix Concatenate4/3, Matrix Concatenate2/3, Matrix Concatenate2/1, Matrix Concatenate6/4, Matrix Concatenate4/4, Matrix Concatenate4/2  "0"
  Demux1/3 -> Matrix Concatenate5/4, Matrix Concatenate6/3  "b1"
  Demux1/4 -> Matrix Concatenate2/4, Matrix Concatenate5/3  "b2"
  Matrix Concatenate14/1 -> Display1/1, M2/1
  Matrix Concatenate13/1 -> Matrix Concatenate14/2
  Matrix Concatenate12/1 -> Matrix Concatenate14/1
  Matrix Concatenate4/1 -> Matrix Concatenate12/1
  Matrix Concatenate5/1 -> Matrix Concatenate13/1
  Matrix Concatenate2/1 -> Matrix Concatenate13/2
  Constant2/1 -> Matrix Concatenate5/2, Matrix Concatenate6/1  "X(2)"
  Constant4/1 -> Matrix Concatenate2/2, Matrix Concatenate5/1  "X(3)"

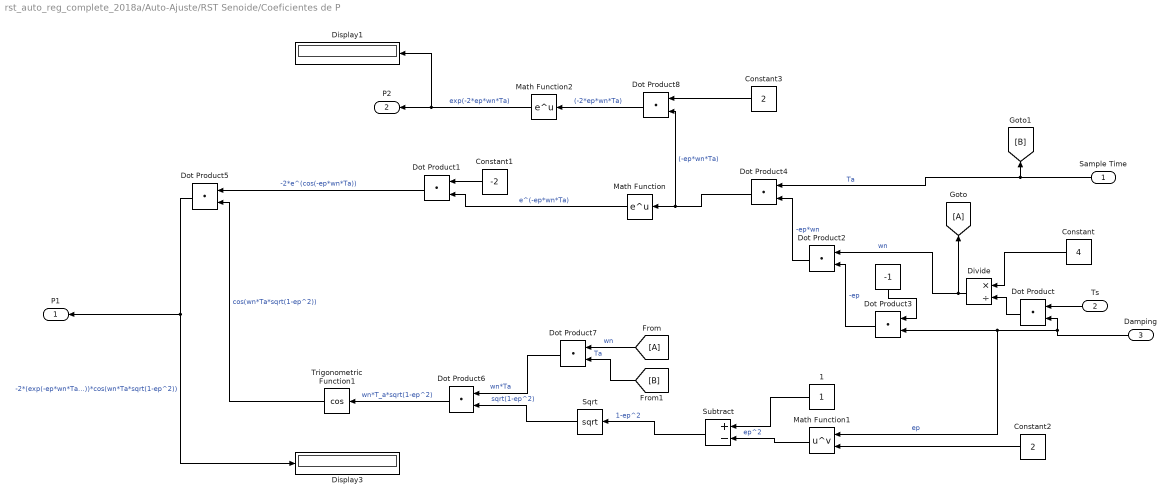
== system rst_auto_reg_complete_2018a/Auto-Ajuste/RST Senoide/Coeficientes de P ==
  Sample Time : Inport
  Ts : Inport  Port=2
  Damping : Inport  Port=3
  " " : Constant  Value=-1
  1 : Constant
  Constant : Constant  Value=4
  Constant1 : Constant  Value=-2
  Constant2 : Constant  Value=2
  Constant3 : Constant  Value=2
  Display1 : Display
  Display3 : Display
  Divide : Product  Inputs=*/
  Dot Product{,1..8} (9 alike) : DotProduct  InputSameDT=on  OutDataTypeStr=Inherit: Inherit via internal rule
  Math Function : Math  SaturateOnIntegerOverflow=on
  Math Function1 : Math  Operator=pow  SaturateOnIntegerOverflow=on
  Math Function2 : Math  SaturateOnIntegerOverflow=on
  Sqrt : Sqrt  SaturateOnIntegerOverflow=on
  Subtract : Sum  Inputs=+-
  Trigonometric Function1 : Trigonometry  Operator=cos
  P1 : Outport
  P2 : Outport  Port=2
  wires:
  Math Function2/1 -> P2/1, Display1/1  "exp(-2*ep*wn*Ta)"
  Dot Product8/1 -> Math Function2/1  "(-2*ep*wn*Ta)"
  Constant3/1 -> Dot Product8/1
  Subtract/1 -> Sqrt/1  "1-ep^2"
  Sqrt/1 -> Dot Product6/2  "sqrt(1-ep^2)"
  Dot Product4/1 -> Math Function/1, Dot Product8/2  "(-ep*wn*Ta)"
  Dot Product6/1 -> Trigonometric Function1/1  "wn*T_a*sqrt(1-ep^2)"
  [B] -> Dot Product7/2  "Ta"
  Dot Product2/1 -> Dot Product4/2  "-ep*wn"
  Constant1/1 -> Dot Product1/1
  1/1 -> Subtract/1
  Constant2/1 -> Math Function1/2
  Dot Product1/1 -> Dot Product5/1  "-2*e^(cos(-ep*wn*Ta))"
  Math Function1/1 -> Subtract/2  "ep^2"
  Sample Time/1 -> [B], Dot Product4/1  "Ta"
  Dot Product7/1 -> Dot Product6/1  "wn*Ta"
  Constant/1 -> Divide/1
  Damping/1 -> Dot Product/2, Dot Product3/2, Math Function1/1  "ep"
  Dot Product3/1 -> Dot Product2/2  "-ep"
  Dot Product/1 -> Divide/2
  Ts/1 -> Dot Product/1
  Trigonometric Function1/1 -> Dot Product5/2  "cos(wn*Ta*sqrt(1-ep^2))"
  Dot Product5/1 -> Display3/1, P1/1  "-2*(exp(-ep*wn*Ta))*cos(wn*Ta*sqrt(1-ep^2))"
  " "/1 -> Dot Product3/1
  [A] -> Dot Product7/1  "wn"
  Divide/1 -> Dot Product2/1, [A]  "wn"
  Math Function/1 -> Dot Product1/2  "e^(-ep*wn*Ta)"

== system rst_auto_reg_complete_2018a/Auto-Ajuste/RST Senoide/Matrix M ==
  In1 : Inport
  " 1" : Constant  Value=0
  2 : Constant
  Demux : Demux
  Display1 : Display
  Matrix Concatenate{6,9..11} (4 alike) : Concatenate  NumInputs=4  Mode=Multidimensional array  ConcatenateDimension=2
  Matrix Concatenate12 : Concatenate  Mode=Multidimensional array
  Matrix Concatenate13 : Concatenate  Mode=Multidimensional array
  Matrix Concatenate14 : Concatenate  Mode=Multidimensional array
  M : Outport
  wires:
  Matrix Concatenate12/1 -> Matrix Concatenate14/1
  Matrix Concatenate13/1 -> Matrix Concatenate14/2
  Matrix Concatenate11/1 -> Matrix Concatenate13/2
  Matrix Concatenate10/1 -> Matrix Concatenate13/1
  Matrix Concatenate9/1 -> Matrix Concatenate12/2
  Matrix Concatenate6/1 -> Matrix Concatenate12/1
  " 1"/1 -> Matrix Concatenate6/2, Matrix Concatenate6/4, Matrix Concatenate9/4, Matrix Concatenate11/1, Matrix Concatenate11/3, Matrix Concatenate6/3  "0"
  2/1 -> Matrix Concatenate6/1, Matrix Concatenate9/2  "1"
  Demux/2 -> Matrix Concatenate10/1, Matrix Concatenate11/2  "a2"
  Demux/4 -> Matrix Concatenate10/3, Matrix Concatenate11/4  "b2"
  Demux/1 -> Matrix Concatenate9/1, Matrix Concatenate10/2  "a1"
  Matrix Concatenate14/1 -> Display1/1, M/1
  Demux/3 -> Matrix Concatenate10/4, Matrix Concatenate9/3  "b1"
  In1/1 -> Demux/1

== system rst_auto_reg_complete_2018a/Auto-Ajuste/RST Senoide/Matrix Q ==
  P1 : Inport
  P2 : Inport  Port=2
  Constant : Constant
  Constant1 : Constant  Value=0
  Display1 : Display
  Matrix Concatenate1 : Concatenate  Mode=Multidimensional array
  Matrix Concatenate2 : Concatenate  Mode=Multidimensional array
  Matrix Concatenate3 : Concatenate  Mode=Multidimensional array
  Q1 : Outport
  wires:
  Constant1/1 -> Matrix Concatenate3/2
  Constant/1 -> Matrix Concatenate1/1
  P1/1 -> Matrix Concatenate1/2
  P2/1 -> Matrix Concatenate3/1
  Matrix Concatenate3/1 -> Matrix Concatenate2/2
  Matrix Concatenate2/1 -> Display1/1, Q1/1
  Matrix Concatenate1/1 -> Matrix Concatenate2/1

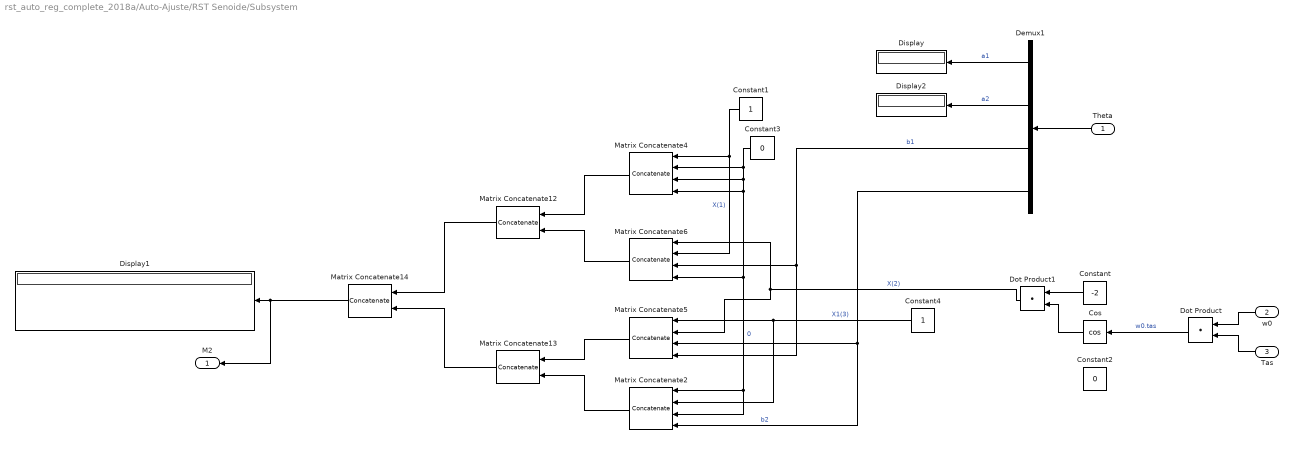
== system rst_auto_reg_complete_2018a/Auto-Ajuste/RST Senoide/Subsystem ==
  Theta : Inport
  w0 : Inport  Port=2
  Tas : Inport  Port=3
  Constant : Constant  Value=-2
  Constant1 : Constant
  Constant2 : Constant  Value=0
  Constant3 : Constant  Value=0
  Constant4 : Constant
  Cos : Trigonometry  Operator=cos
  Demux1 : Demux
  Display : Display
  Display1 : Display
  Display2 : Display
  Dot Product : DotProduct  InputSameDT=on  OutDataTypeStr=Inherit: Inherit via internal rule
  Dot Product1 : DotProduct  InputSameDT=on  OutDataTypeStr=Inherit: Inherit via internal rule
  Matrix Concatenate12 : Concatenate  Mode=Multidimensional array
  Matrix Concatenate13 : Concatenate  Mode=Multidimensional array
  Matrix Concatenate14 : Concatenate  Mode=Multidimensional array
  Matrix Concatenate{2,4..6} (4 alike) : Concatenate  NumInputs=4  Mode=Multidimensional array  ConcatenateDimension=2
  M2 : Outport
  wires:
  Constant/1 -> Dot Product1/1
  Cos/1 -> Dot Product1/2
  Matrix Concatenate6/1 -> Matrix Concatenate12/2
  Demux1/2 -> Display2/1  "a2"
  Dot Product/1 -> Cos/1  "w0.tas"
  Tas/1 -> Dot Product/2
  w0/1 -> Dot Product/1
  Theta/1 -> Demux1/1
  Demux1/1 -> Display/1  "a1"
  Constant1/1 -> Matrix Concatenate6/2, Matrix Concatenate4/1  "X(1)"
  Constant3/1 -> Matrix Concatenate4/3, Matrix Concatenate2/3, Matrix Concatenate2/1, Matrix Concatenate6/4, Matrix Concatenate4/4, Matrix Concatenate4/2  "0"
  Dot Product1/1 -> Matrix Concatenate5/2, Matrix Concatenate6/1  "X(2)"
  Constant4/1 -> Matrix Concatenate2/2, Matrix Concatenate5/1  "X1(3)"
  Demux1/3 -> Matrix Concatenate5/4, Matrix Concatenate6/3  "b1"
  Demux1/4 -> Matrix Concatenate2/4, Matrix Concatenate5/3  "b2"
  Matrix Concatenate14/1 -> Display1/1, M2/1
  Matrix Concatenate13/1 -> Matrix Concatenate14/2
  Matrix Concatenate12/1 -> Matrix Concatenate14/1
  Matrix Concatenate4/1 -> Matrix Concatenate12/1
  Matrix Concatenate5/1 -> Matrix Concatenate13/1
  Matrix Concatenate2/1 -> Matrix Concatenate13/2
